simulink library "vmc"  (R2021b)
settings: Solver=VariableStepAuto  StartTime=0.0  StopTime=10.0  RelTol=1e-3
undefined symbols (not defined in the file or in its folder): AVMC_ACCDeltaTqIGain_X_kph, AVMC_ACCDeltaTqIGain_Y_mps2, AVMC_ACCDeltaTqPGain_X_kph, AVMC_ACCDeltaTqPGain_Y_kph, AVMC_ACCLongSteadyCtrl_X_kph, AVMC_AggressJerkPCT4AT_X_kph, AVMC_AggressJerkPCT_X_kph, AVMC_AggressLimitPCT4AT_X_kph, AVMC_AggressLimitPCT_X_kph, AVMC_CCLongSteadyCtrl_X_kph, AVMC_DISCDeltaTqIGain_X_kph, AVMC_DISCDeltaTqIGain_Y_mps2, AVMC_DISCDeltaTqPGain_X_kph, AVMC_DISCDeltaTqPGain_Y_kph, AVMC_DISCTrunAccJerk_X_s, AVMC_DISCTrunAccLimit_X_s, AVMC_ESCRegenOut_X_kph, AVMC_ESCRegenOut_Y_Deg, AVMC_ESCRegenOutEnSpd_X_Deg, AVMC_ISOAccLimit_X_mps, AVMC_ISODecLimit_X_mps, AVMC_ISOJerk_X_mps, AVMC_LatESCRegenOut_X_kph, AVMC_LatESCRegenOut_Y_Deg, AVMC_LongAccDeadZone_X_kph, AVMC_LongAccFiltTsforP2_X_Gps, AVMC_MCPresBaseTq_X_bar, AVMC_MSALongSteadyCtrl_X_kph, AVMC_MSAPedalOvrd2_X_kph, AVMC_MSAPedalOvrd_X_kph, AVMC_MSASpdBand_X_kph, AVMC_MSATqDownEndTq_X_kph, AVMC_MSATqDownTime_X_kph, AVMC_RDCDetectTime_X_kph, AVMC_RDCDetectTime_Y_pct, AVMC_RDCEnSlideRate_X_Deg, AVMC_RearWhlTqRatio_X_Nm, AVMC_RearWhlTqRatio_Y_gps, AVMC_RearWhlTqSlipGain_X_rat, AVMC_RearWhlTqSlipGain_Y_kph, AVMC_SoftJerkPCT_X_kph, AVMC_SoftLimitPCT_X_kph, AVMC_StESCYaw_X_kph, AVMC_StESCYaw_Y_Deg, AVMC_StESCYawCom_X_kph, AVMC_StESCYawCom_Y_Gps, AVMC_TMSpdBaseTq_X_rpm, AVMC_VehHoldBDecMap_X_kph, AVMC_VehHoldDecCtrlTime_X_kph, AVMC_VehHoldMCPPass_X_deg, C_TASK_10MS_S, C_TASK_5MS_S, DEG2RAD, Discrete, ENUM_ACCAVAIL_AVAILABLE, ENUM_ACCCTRLALLOW_ALLOW, ENUM_ADASACCSTA_ACTIVE, ENUM_ADASACCSTA_OVERRIDE, ENUM_ADASACCSTA_SHUTOFF, ENUM_ADASAEBREQ_NOREQUEST ... (+361)
libraries: hcu_lib x63, simulink x60, simulink_extras x3, ctrlSharedLib x3, $bdroot x2
(part 4 of 15)

== system vmc/VMC/VMC/PreConditionCheck ==
  VINP_DriverSeatBeltCmd_flg : Inport
  VBCM_DrDoorSW_flg : Inport  Port=2
  VTQD_GearActualPosn_enum : Inport  Port=3
  VINP_BrkSwSta_flg : Inport  Port=4
  VINP_EPBSta_enum : Inport  Port=5
  VINP_ACCAvail_flg : Inport  Port=6
  VINP_AEBAvail_flg : Inport  Port=7
  VINP_ESCOFFStatus_enum : Inport  Port=8
  VAPS_APSStaSystem_enum : Inport  Port=9
  VTQD_ExternalTqAllow_flg : Inport  Port=10
  VVMC_ACCCtrlAvail_flg : Inport  Port=11
  task_time_s : Inport  Port=12
  VINP_BrkPedalPos_pct : Inport  Port=13
  Cast To Single : DataTypeConversion  OutDataTypeStr=boolean
  Constant : Constant  Value=ENUM_DRDOORSW_CLOSE
  Constant1 : Constant  Value=ENUM_GEARACTUALPOSN_D
  Constant10 : Constant  Value=ENUM_APSSTASYSTEM_ACTIVE
  Constant11 : Constant  Value=ENUM_APSSTASYSTEM_REMOTEACTIVE
  Constant12 : Constant  Value=ENUM_EXTERNALTQALLOW_ALLOW
  Constant13 : Constant  Value=ENUM_ACCCTRLALLOW_ALLOW
  Constant14 : Constant  Value=ENUM_DRDOORSW_CLOSE
  Constant15 : Constant  Value=ENUM_GEARACTUALPOSN_D
  Constant16 : Constant  Value=KVMC_APSSWC_flg
  Constant17 : Constant  Value=ENUM_EPBSTA_RELEASED
  Constant18 : Constant  Value=ENUM_EXTERNALTQALLOW_ALLOW
  Constant{19,21,24,27,30} (5 alike) : Constant  Value=TRUE
  Constant2 : Constant  Value=ENUM_BRKSWSTA_INACTIVE
  Constant{20,23,26,29} (4 alike) : Constant  Value=KVMC_PreCheckAllowTime_s
  Constant{22,25,28,31} (4 alike) : Constant  Value=FALSE
  Constant3 : Constant  Value=ENUM_EPBSTA_RELEASED
  Constant32 : Constant  Value=KVMC_BrkEnBand_pct
  Constant33 : Constant  Value=KVMC_BrkPreCheckSW_flg
  Constant4 : Constant  Value=ENUM_ACCAVAIL_AVAILABLE
  Constant5 : Constant  Value=ENUM_AEBAVAIL_AVAILABLE
  Constant6 : Constant  Value=ENUM_ESCOFFSTATUS_NORMAL
  Constant7 : Constant  Value=ENUM_DRIVERSEATBELTCMD_LAMPOFF
  Constant8 : Constant  Value=ENUM_GEARACTUALPOSN_D
  Constant9 : Constant  Value=ENUM_GEARACTUALPOSN_N
  Logical Operator : Logic  AllPortsSameDT=off  OutDataTypeStr=boolean
  Logical Operator1 : Logic  Inputs=6  AllPortsSameDT=off  OutDataTypeStr=boolean
  Logical Operator2 : Logic  Inputs=3  AllPortsSameDT=off  OutDataTypeStr=boolean
  Logical Operator3 : Logic  Inputs=3  AllPortsSameDT=off  OutDataTypeStr=boolean
  Logical Operator4 : Logic  AllPortsSameDT=off  OutDataTypeStr=boolean
  Logical Operator5 : Logic  Inputs=4  AllPortsSameDT=off  OutDataTypeStr=boolean
  Logical Operator6 : Logic  Operator=OR  AllPortsSameDT=off  OutDataTypeStr=boolean
  NOT{,1..3} (4 alike) : Logic  Operator=NOT  AllPortsSameDT=off  OutDataTypeStr=boolean
  Relational Operator{,1..9,12..15,17..18} (16 alike) : RelationalOperator  Operator===  OutDataTypeStr=boolean  RndMeth=Simplest
  Relational Operator10 : RelationalOperator  Operator=~=  OutDataTypeStr=boolean  RndMeth=Simplest
  Relational Operator11 : RelationalOperator  Operator=~=  OutDataTypeStr=boolean  RndMeth=Simplest
  Relational Operator{16,19..21} (4 alike) : RelationalOperator  OutDataTypeStr=boolean  RndMeth=Simplest
  Relational Operator22 : RelationalOperator  Operator=<=  OutDataTypeStr=boolean  RndMeth=Simplest
  Switch : Switch  Criteria=u2 > Threshold
  Timer{,1..3} (4 alike) : hcu_lib/Basic_Blocks/Timer
  u2 > 0 : Switch  Criteria=u2 > Threshold
  u2 > 0 (1){,1..3} (4 alike) : Switch  Criteria=u2 > Threshold
  VVMC_VMCACCCtrlAvail_flg : Outport
  VVMC_VMCAEBCtrlAvail_flg : Outport  Port=2
  VVMC_VMCCCCtrlAvail_flg : Outport  Port=3
  VVMC_VMCMSACtrlAvail_flg : Outport  Port=4
  wires:
  [task_time_s] -> Timer3/3
  Constant31/1 -> u2 > 0 (1)3/3
  Relational Operator21/1 -> u2 > 0 (1)3/2
  Timer3/1 -> Relational Operator21/1
  Constant29/1 -> Relational Operator21/2, Timer3/4
  Constant30/1 -> u2 > 0 (1)3/1
  Logical Operator5/1 -> NOT3/1, Timer3/1
  NOT3/1 -> Timer3/2
  u2 > 0 (1)3/1 -> [VVMC_VMCMSACtrlAvail_flg]  "VVMC_VMCMSACtrlAvail_flg"
  u2 > 0 (1)2/1 -> [VVMC_VMCCCCtrlAvail_flg]  "VVMC_VMCCCCtrlAvail_flg"
  NOT2/1 -> Timer2/2
  Logical Operator4/1 -> Timer2/1, NOT2/1
  Constant27/1 -> u2 > 0 (1)2/1
  Constant26/1 -> Timer2/4, Relational Operator20/2
  Timer2/1 -> Relational Operator20/1
  Relational Operator20/1 -> u2 > 0 (1)2/2
  Constant28/1 -> u2 > 0 (1)2/3
  [task_time_s] -> Timer2/3
  u2 > 0 (1)1/1 -> [VVMC_VMCACCCtrlAvail_flg]  "VVMC_VMCACCCtrlAvail_flg"
  [task_time_s] -> Timer1/3
  Constant25/1 -> u2 > 0 (1)1/3
  Relational Operator19/1 -> u2 > 0 (1)1/2
  Timer1/1 -> Relational Operator19/1
  Constant23/1 -> Relational Operator19/2, Timer1/4
  Constant24/1 -> u2 > 0 (1)1/1
  Logical Operator2/1 -> NOT1/1, Timer1/1
  NOT1/1 -> Timer1/2
  task_time_s/1 -> [task_time_s]
  u2 > 0 (1)/1 -> [VVMC_VMCAEBCtrlAvail_flg]  "VVMC_VMCAEBCtrlAvail_flg"
  Logical Operator3/1 -> NOT/1, Timer/1
  NOT/1 -> Timer/2
  Constant21/1 -> u2 > 0 (1)/1
  Constant20/1 -> Relational Operator16/2, Timer/4
  Relational Operator16/1 -> u2 > 0 (1)/2
  Timer/1 -> Relational Operator16/1
  [task_time_s] -> Timer/3
  Constant22/1 -> u2 > 0 (1)/3
  Cast To Single/1 -> Logical Operator1/6
  u2 > 0/1 -> Cast To Single/1
  Constant19/1 -> u2 > 0/3
  Constant16/1 -> u2 > 0/2
  Relational Operator5/1 -> Logical Operator3/3
  Relational Operator7/1 -> Logical Operator3/1
  Logical Operator6/1 -> Logical Operator3/2
  Relational Operator8/1 -> Logical Operator6/1
  Relational Operator9/1 -> Logical Operator6/2
  [VTQD_GearActualPosn_enum] -> Relational Operator9/1  "VTQD_GearActualPosn_enum"
  Constant9/1 -> Relational Operator9/2
  Constant8/1 -> Relational Operator8/2
  [VTQD_GearActualPosn_enum] -> Relational Operator8/1  "VTQD_GearActualPosn_enum"
  Constant7/1 -> Relational Operator7/2
  [VINP_DriverSeatBeltCmd_flg] -> Relational Operator7/1
  VINP_DriverSeatBeltCmd_flg/1 -> [VINP_DriverSeatBeltCmd_flg]
  [VVMC_VMCMSACtrlAvail_flg] -> VVMC_VMCMSACtrlAvail_flg/1
  Relational Operator18/1 -> Logical Operator5/4
  Relational Operator17/1 -> Logical Operator5/3
  Relational Operator15/1 -> Logical Operator5/2
  Relational Operator14/1 -> Logical Operator5/1
  Constant18/1 -> Relational Operator18/2
  [VTQD_ExternalTqAllow_flg] -> Relational Operator18/1
  Constant14/1 -> Relational Operator14/2
  [VBCM_DrDoorSW_flg] -> Relational Operator14/1  "VBCM_DrDoorSW_flg"
  Constant15/1 -> Relational Operator15/2
  [VTQD_GearActualPosn_enum] -> Relational Operator15/1  "VTQD_GearActualPosn_enum"
  Constant17/1 -> Relational Operator17/2
  [VINP_EPBSta_enum] -> Relational Operator17/1  "VINP_EPBSta_enum"
  Relational Operator13/1 -> Logical Operator2/2
  [VVMC_ACCCtrlAvail_flg] -> Relational Operator13/1
  Constant13/1 -> Relational Operator13/2
  VVMC_ACCCtrlAvail_flg/1 -> [VVMC_ACCCtrlAvail_flg]
  [VVMC_VMCCCCtrlAvail_flg] -> VVMC_VMCCCCtrlAvail_flg/1
  Relational Operator12/1 -> Logical Operator4/2
  [VTQD_ExternalTqAllow_flg] -> Relational Operator12/1
  Constant12/1 -> Relational Operator12/2
  VTQD_ExternalTqAllow_flg/1 -> [VTQD_ExternalTqAllow_flg]
  [VVMC_VMCACCCtrlAvail_flg] -> VVMC_VMCACCCtrlAvail_flg/1
  [VVMC_VMCAEBCtrlAvail_flg] -> VVMC_VMCAEBCtrlAvail_flg/1
  Logical Operator1/1 -> Logical Operator4/1, Logical Operator2/3
  Relational Operator4/1 -> Logical Operator2/1
  Logical Operator/1 -> u2 > 0/1
  Relational Operator6/1 -> Logical Operator1/5
  Relational Operator3/1 -> Logical Operator1/4
  Switch/1 -> Logical Operator1/3
  Relational Operator1/1 -> Logical Operator1/2
  Relational Operator/1 -> Logical Operator1/1
  Relational Operator11/1 -> Logical Operator/2
  Relational Operator10/1 -> Logical Operator/1
  Constant11/1 -> Relational Operator11/2
  [VAPS_APSStaSystem_enum] -> Relational Operator11/1  "VAPS_APSStaSystem_enum"
  Constant10/1 -> Relational Operator10/2
  [VAPS_APSStaSystem_enum] -> Relational Operator10/1  "VAPS_APSStaSystem_enum"
  Constant6/1 -> Relational Operator6/2
  [VINP_ESCOFFStatus_enum] -> Relational Operator6/1  "VINP_ESCOFFStatus_enum"
  Constant5/1 -> Relational Operator5/2
  [VINP_AEBAvail_flg] -> Relational Operator5/1  "VINP_AEBAvail_flg"
  Constant4/1 -> Relational Operator4/2
  [VINP_ACCAvail_flg] -> Relational Operator4/1  "VINP_ACCAvail_flg"
  [VINP_EPBSta_enum] -> Relational Operator3/1  "VINP_EPBSta_enum"
  Constant3/1 -> Relational Operator3/2
  Constant2/1 -> Relational Operator2/2
  [VINP_BrkSwSta_flg] -> Relational Operator2/1  "VINP_BrkSwSta_flg"
  [VTQD_GearActualPosn_enum] -> Relational Operator1/1  "VTQD_GearActualPosn_enum"
  Constant1/1 -> Relational Operator1/2
  [VBCM_DrDoorSW_flg] -> Relational Operator/1  "VBCM_DrDoorSW_flg"
  Constant/1 -> Relational Operator/2
  VAPS_APSStaSystem_enum/1 -> [VAPS_APSStaSystem_enum]
  VINP_ESCOFFStatus_enum/1 -> [VINP_ESCOFFStatus_enum]
  VINP_AEBAvail_flg/1 -> [VINP_AEBAvail_flg]
  VINP_ACCAvail_flg/1 -> [VINP_ACCAvail_flg]
  VINP_EPBSta_enum/1 -> [VINP_EPBSta_enum]
  VINP_BrkSwSta_flg/1 -> [VINP_BrkSwSta_flg]
  VTQD_GearActualPosn_enum/1 -> [VTQD_GearActualPosn_enum]
  VBCM_DrDoorSW_flg/1 -> [VBCM_DrDoorSW_flg]
  VINP_BrkPedalPos_pct/1 -> [VINP_BrkPedalPos_pct]
  Constant32/1 -> Relational Operator22/2
  Constant33/1 -> Switch/2
  Relational Operator22/1 -> Switch/1
  [VINP_BrkPedalPos_pct] -> Relational Operator22/1
  Relational Operator2/1 -> Switch/3

== system vmc/VMC/VMC/RDC Determination ==
  task_time_s : Inport
  VVMC_ActMaxSlideRate_pct : Inport  Port=2
  VTQD_AfterAvailableTqDemFr_Nm : Inport  Port=3
  VTQD_AfterAvailableTqDemRr_Nm : Inport  Port=4
  VINP_ESCActive_flg : Inport  Port=5
  VINP_SASAngle_Deg : Inport  Port=6
  VINP_LatAccel_Gps : Inport  Port=7
  VINP_VehSpeed_kph : Inport  Port=8
  VINP_YawRate_degps : Inport  Port=9
  VINP_RDCActive_enum : Inport  Port=10
  VINP_DIDGetDynoMode_flg : Inport  Port=11
  RWD : Subsystem
  VVMC_RWDRDCActive_enum : Outport
  VVMC_RDCEnSlideRate_pct : Outport  Port=2
  VVMC_ActStESCYaw_degps : Outport  Port=3
  wires:
  [VINP_YawRate_degps] -> RWD/9(VINP_YawRate_degps)
  VTQD_AfterAvailableTqDemFr_Nm/1 -> [VTQD_AfterAvailableTqDemFr_Nm]
  [VTQD_AfterAvailableTqDemRr_Nm] -> RWD/4(VTQD_AfterAvailableTqDemRr_Nm)
  [VINP_RDCActive_enum] -> RWD/10(VINP_RDCActive_enum)
  [VINP_VehSpeed_kph] -> RWD/8(VINP_VehSpeed_kph)
  [VVMC_RWDRDCActive_enum] -> VVMC_RWDRDCActive_enum/1
  [VINP_LatAccel_Gps] -> RWD/7(VINP_LatAccel_Gps)
  [VVMC_ActMaxSlideRate_pct] -> RWD/2(VVMC_ActMaxSlideRate_pct)
  [VINP_SASAngle_Deg] -> RWD/6(VINP_SASAngle_Deg)
  [task_time_s] -> RWD/1(task_time_s)
  [VTQD_AfterAvailableTqDemFr_Nm] -> RWD/3(VTQD_AfterAvailableTqDemFr_Nm)
  [VINP_ESCActive_flg] -> RWD/5(VINP_ESCActive_flg)
  VINP_RDCActive_enum/1 -> [VINP_RDCActive_enum]
  VINP_SASAngle_Deg/1 -> [VINP_SASAngle_Deg]
  VTQD_AfterAvailableTqDemRr_Nm/1 -> [VTQD_AfterAvailableTqDemRr_Nm]
  task_time_s/1 -> [task_time_s]
  VVMC_ActMaxSlideRate_pct/1 -> [VVMC_ActMaxSlideRate_pct]
  VINP_LatAccel_Gps/1 -> [VINP_LatAccel_Gps]
  VINP_ESCActive_flg/1 -> [VINP_ESCActive_flg]
  VINP_VehSpeed_kph/1 -> [VINP_VehSpeed_kph]
  VINP_YawRate_degps/1 -> [VINP_YawRate_degps]
  RWD/1(VVMC_RWDRDCActive_enum) -> [VVMC_RWDRDCActive_enum]
  RWD/2(VVMC_RDCEnSlideRate_pct) -> [VVMC_RDCEnSlideRate_pct]
  RWD/3(VVMC_ActStESCYaw_Dps) -> [VVMC_ActStESCYaw_degps]
  [VVMC_RDCEnSlideRate_pct] -> VVMC_RDCEnSlideRate_pct/1
  [VVMC_ActStESCYaw_degps] -> VVMC_ActStESCYaw_degps/1
  VINP_DIDGetDynoMode_flg/1 -> [VINP_DIDGetDynoMode_flg]
  [VINP_DIDGetDynoMode_flg] -> RWD/11(VINP_DIDGetDynoMode_flg)

== system vmc/VMC/VMC/SPD2ACC ==
  VVMC_FeatArbitrSta_enum : Inport
  VINP_ADASACCSta_enum : Inport  Port=2
  VVMC_FeatReqSpd_kph : Inport  Port=3
  VVMC_LimitPCT_pct : Inport  Port=4
  VVMC_JerkPCT_pct : Inport  Port=5
  VINP_VehSpeed_kph : Inport  Port=6
  VVMC_MeterIndSpeedForCalcu_kph : Inport  Port=7
  VVMC_SafetyCtrl_flg : Inport  Port=8
  VINP_ACCRequiredAccel_mps2 : Inport  Port=9
  task_time_s : Inport  Port=10
  VVMC_LongAcc_Gps : Inport  Port=11
  VINP_ESCADASSta_enum : Inport  Port=12
  VVMC_LastADASWhlTqReq_Nm : Inport  Port=13
  VTQD_RrEDUAvailBrkRgnTq_Nm : Inport  Port=14
  VVMC_ACCVehHoldReq_flg : Inport  Port=15
  VVMC_EstSlope_Deg : Inport  Port=16
  VVMC_LongAccDeadZone_Gps : Inport  Port=17
  VTQD_FrEDUAvailBrkRgnTq_Nm : Inport  Port=18
  VVMC_ACCLowSpdTqCtrl_flg : Inport  Port=19
  VDSC_DISCTurn_flg : Inport  Port=20
  VINP_GRADE_Deg : Inport  Port=21
  VINP_LFWhlRotDir_enum : Inport  Port=22
  VINP_LRWhlRotDir_enum : Inport  Port=23
  VINP_RFWhlRotDir_enum : Inport  Port=24
  VINP_RRWhlRotDir_enum : Inport  Port=25
  VVMC_ACCObjDist_m : Inport  Port=26
  VINP_MCPressure_bar : Inport  Port=27
  VVMC_AccelTurnHold_flg : Inport  Port=28
  Cast To Boolean : DataTypeConversion  OutDataTypeStr=boolean
  Cast To Boolean1 : DataTypeConversion  OutDataTypeStr=boolean
  Cast To Single : DataTypeConversion  OutDataTypeStr=boolean
  Cast To Single{1..2,4..7,9} (7 alike) : DataTypeConversion  OutDataTypeStr=single
  Cast To Single8 : DataTypeConversion  OutDataTypeStr=uint8
  ISO22179 : Subsystem
  PID : Subsystem
  ReqACCCalcu : Subsystem
  SPD2ACC Active Determination : Subsystem
  VVMC_ACCRequiredAccel_mps2 : Outport
  VVMC_DISCReqAcc_mps2 : Outport  Port=2
  VVMC_FeatArbitrFinal_enum : Outport  Port=3
  VVMC_SPD2ACCAct_flg : Outport  Port=4
  VVMC_AccCalcuPID_mps2 : Outport  Port=5
  VVMC_ISOAccLimit_mps2 : Outport  Port=6
  VVMC_ISODecLimit_mps2 : Outport  Port=7
  VVMC_ISOJerkLimit_mps3 : Outport  Port=8
  VVMC_VehHoldReq_flg : Outport  Port=9
  VVMC_ActACCRequiredAccel_mps2 : Outport  Port=10
  VVMC_VehHoldDecCtrlHEnd_flg : Outport  Port=11
  wires:
  [task_time_s] -> ReqACCCalcu/13(task_time_s)
  task_time_s/1 -> [task_time_s]
  [VINP_VehSpeed_kph] -> PID/3(VINP_VehSpeed_kph)
  VINP_VehSpeed_kph/1 -> [VINP_VehSpeed_kph]
  [VVMC_ISOJerkLimit_mps3] -> VVMC_ISOJerkLimit_mps3/1
  [VVMC_ISODecLimit_mps2] -> VVMC_ISODecLimit_mps2/1
  [VVMC_ISOAccLimit_mps2] -> VVMC_ISOAccLimit_mps2/1
  [VVMC_AccCalcuPID_mps2] -> VVMC_AccCalcuPID_mps2/1
  [VVMC_SPD2ACCAct_flg] -> VVMC_SPD2ACCAct_flg/1
  [VVMC_FeatReqSpd_kph] -> ReqACCCalcu/12(VVMC_FeatReqSpd_kph)
  [VVMC_MeterIndSpeedForCalcu_kph] -> ReqACCCalcu/11(VVMC_MeterIndSpeedForCalcu_kph)
  [VINP_ADASACCSta_enum] -> ReqACCCalcu/10(VINP_ADASACCSta_enum)
  VINP_ADASACCSta_enum/1 -> [VINP_ADASACCSta_enum]
  [VVMC_ActACCRequiredAccel_mps2] -> VVMC_DISCReqAcc_mps2/1  "VVMC_DISCReqAcc_mps2"
  [VVMC_FeatArbitrFinal_enum] -> VVMC_FeatArbitrFinal_enum/1
  Cast To Single8/1 -> [VVMC_FeatArbitrFinal_enum]  "VVMC_FeatArbitrFinal_enum"
  ReqACCCalcu/2(VVMC_FeatArbitrFinal_enum) -> Cast To Single8/1
  [VVMC_FeatArbitrSta_enum] -> ReqACCCalcu/9(VVMC_FeatArbitrSta_enum)
  [VINP_ACCRequiredAccel_mps2] -> ReqACCCalcu/8(VINP_ACCRequiredAccel_mps2)
  VINP_ACCRequiredAccel_mps2/1 -> [VINP_ACCRequiredAccel_mps2]
  VVMC_SafetyCtrl_flg/1 -> [VVMC_SafetyCtrl_flg]
  [VVMC_SafetyCtrl_flg] -> ReqACCCalcu/7(VVMC_SafetyCtrl_flg)
  Cast To Single7/1 -> [VVMC_ACCRequiredAccel_mps2]  "VVMC_ACCRequiredAccel_mps2"
  Cast To Single6/1 -> [VVMC_ISOJerkLimit_mps3]  "VVMC_ISOJerkLimit_mps3"
  Cast To Single5/1 -> [VVMC_ISODecLimit_mps2]  "VVMC_ISODecLimit_mps2"
  Cast To Single4/1 -> [VVMC_ISOAccLimit_mps2]  "VVMC_ISOAccLimit_mps2"
  Cast To Single2/1 -> [VVMC_MeterSpdCalcu_mps]  "VVMC_MeterSpdCalcu_mps"
  Cast To Single1/1 -> [VVMC_AccCalcuPID_mps2]  "VVMC_AccCalcuPID_mps2"
  Cast To Single/1 -> [VVMC_SPD2ACCAct_flg]  "VVMC_SPD2ACCAct_flg"
  [VVMC_ACCRequiredAccel_mps2] -> VVMC_ACCRequiredAccel_mps2/1
  ReqACCCalcu/1("VVMC_ACCRequiredAccel_mps2 ") -> Cast To Single7/1
  [VVMC_SPD2ACCAct_flg] -> ReqACCCalcu/6(VVMC_SPD2ACCAct_flg)
  PID/2(VVMC_MeterSpdCalcu_mps) -> Cast To Single2/1
  PID/1(VVMC_AccCalcuPID_mps2) -> Cast To Single1/1
  [VVMC_FeatReqSpd_kph] -> PID/2(VVMC_FeatReqSpd_kph)
  [VVMC_MeterIndSpeedForCalcu_kph] -> PID/4(VVMC_MeterIndSpeedForCalcu_kph)
  [VVMC_SPD2ACCAct_flg] -> PID/1(VVMC_SPD2ACCAct_flg)
  ISO22179/3(VVMC_ISOJerkLimit_mps3) -> Cast To Single6/1
  [VVMC_MeterSpdCalcu_mps] -> ISO22179/1(VVMC_MeterSpdCalcu_mps)
  ISO22179/2(VVMC_ISODecLimit_mps2) -> Cast To Single5/1
  ISO22179/1(VVMC_ISOAccLimit_mps2) -> Cast To Single4/1
  [VVMC_LimitPCT_pct] -> ISO22179/2(VVMC_LimitPCT_pct)
  SPD2ACC Active Determination/1(VVMC_SPD2ACCAct_flg) -> Cast To Single/1
  [VVMC_FeatArbitrSta_enum] -> SPD2ACC Active Determination/1(VVMC_FeatArbitrSta_enum)
  VVMC_FeatArbitrSta_enum/1 -> [VVMC_FeatArbitrSta_enum]
  VVMC_MeterIndSpeedForCalcu_kph/1 -> [VVMC_MeterIndSpeedForCalcu_kph]
  VVMC_LimitPCT_pct/1 -> [VVMC_LimitPCT_pct]
  VVMC_JerkPCT_pct/1 -> [VVMC_JerkPCT_pct]
  VVMC_FeatReqSpd_kph/1 -> [VVMC_FeatReqSpd_kph]
  [VVMC_JerkPCT_pct] -> ReqACCCalcu/3(VVMC_JerkPCT_pct)
  [VVMC_ISOJerkLimit_mps3] -> ReqACCCalcu/2(VVMC_ISOJerkLimit_mps3)
  [VVMC_AccCalcuPID_mps2] -> ReqACCCalcu/1(VVMC_AccCalcuPID_mps2)
  [VVMC_ISOAccLimit_mps2] -> ReqACCCalcu/4(VVMC_ISOAccLimit_mps2)
  [VVMC_ISODecLimit_mps2] -> ReqACCCalcu/5(VVMC_ISODecLimit_mps2)
  [VINP_VehSpeed_kph] -> ReqACCCalcu/14(VINP_VehSpeed_kph)
  [VVMC_LongAcc_Gps] -> ReqACCCalcu/15(VVMC_LongAcc_Gps)
  VVMC_LongAcc_Gps/1 -> [VVMC_LongAcc_Gps]
  [VTQD_RrEDUAvailBrkRgnTq_Nm] -> ReqACCCalcu/18(VTQD_RrEDUAvailBrkRgnTq_Nm)
  [VVMC_LastADASWhlTqReq_Nm] -> ReqACCCalcu/17(VVMC_LastADASWhlTqReq_Nm)
  [VINP_ESCADASSta_enum] -> ReqACCCalcu/16(VINP_ESCADASSta_enum)
  Cast To Boolean/1 -> [VVMC_VehHoldReq_flg]  "VVMC_VehHoldReq_flg"
  Cast To Single9/1 -> [VVMC_ActACCRequiredAccel_mps2]  "VVMC_ActACCRequiredAccel_mps2"
  ReqACCCalcu/4(VVMC_ActACCRequiredAccel_mps2) -> Cast To Single9/1
  ReqACCCalcu/3(VVMC_VehHoldReq_flg) -> Cast To Boolean/1
  VTQD_RrEDUAvailBrkRgnTq_Nm/1 -> [VTQD_RrEDUAvailBrkRgnTq_Nm]
  VINP_ESCADASSta_enum/1 -> [VINP_ESCADASSta_enum]
  VVMC_LastADASWhlTqReq_Nm/1 -> [VVMC_LastADASWhlTqReq_Nm]
  [VVMC_ActACCRequiredAccel_mps2] -> VVMC_ActACCRequiredAccel_mps2/1
  [VVMC_VehHoldReq_flg] -> VVMC_VehHoldReq_flg/1  "VVMC_VehHoldReq_flg"
  VVMC_ACCVehHoldReq_flg/1 -> [VVMC_ACCVehHoldReq_flg]
  [VVMC_ACCVehHoldReq_flg] -> ReqACCCalcu/19(VVMC_ACCVehHoldReq_flg)
  VVMC_EstSlope_Deg/1 -> [VVMC_EstSlope_Deg]
  [VVMC_EstSlope_Deg] -> ReqACCCalcu/20(VVMC_EstSlope_Deg)
  VVMC_LongAccDeadZone_Gps/1 -> [VVMC_LongAccDeadZone_Gps]
  [VVMC_LongAccDeadZone_Gps] -> ReqACCCalcu/21(VVMC_LongAccDeadZone_Gps)
  ReqACCCalcu/5(VVMC_VehHoldDecCtrlHEnd_flg) -> Cast To Boolean1/1
  Cast To Boolean1/1 -> [VVMC_VehHoldDecCtrlHEnd_flg]
  [VVMC_VehHoldDecCtrlHEnd_flg] -> VVMC_VehHoldDecCtrlHEnd_flg/1
  VTQD_FrEDUAvailBrkRgnTq_Nm/1 -> [VTQD_FrEDUAvailBrkRgnTq_Nm]
  [VTQD_FrEDUAvailBrkRgnTq_Nm] -> ReqACCCalcu/22(VTQD_FrEDUAvailBrkRgnTq_Nm)
  VVMC_ACCLowSpdTqCtrl_flg/1 -> [VVMC_ACCLowSpdTqCtrl_flg]
  [VVMC_ACCLowSpdTqCtrl_flg] -> ReqACCCalcu/23(VVMC_ACCLowSpdTqCtrl_flg)
  VDSC_DISCTurn_flg/1 -> [VDSC_DISCTurn_flg]
  [VDSC_DISCTurn_flg] -> ReqACCCalcu/24(VDSC_DISCTurn_flg)
  VINP_GRADE_Deg/1 -> [VINP_GRADE_Deg]
  [VINP_GRADE_Deg] -> ReqACCCalcu/25(VINP_GRADE_Deg)
  VINP_LRWhlRotDir_enum/1 -> [VINP_LRWhlRotDir_enum]
  VINP_RFWhlRotDir_enum/1 -> [VINP_RFWhlRotDir_enum]
  VINP_LFWhlRotDir_enum/1 -> [VINP_LFWhlRotDir_enum]
  VINP_RRWhlRotDir_enum/1 -> [VINP_RRWhlRotDir_enum]
  [VINP_RRWhlRotDir_enum] -> ReqACCCalcu/29(VINP_RRWhlRotDir_enum)
  [VINP_RFWhlRotDir_enum] -> ReqACCCalcu/28(VINP_RFWhlRotDir_enum)
  [VINP_LRWhlRotDir_enum] -> ReqACCCalcu/27(VINP_LRWhlRotDir_enum)
  [VINP_LFWhlRotDir_enum] -> ReqACCCalcu/26(VINP_LFWhlRotDir_enum)
  VVMC_ACCObjDist_m/1 -> [VVMC_ACCObjDist_m]
  [VVMC_ACCObjDist_m] -> ReqACCCalcu/30(VVMC_ACCObjDist_m)
  VINP_MCPressure_bar/1 -> [VINP_MCPressure_bar]
  [VINP_MCPressure_bar] -> ReqACCCalcu/31(VINP_MCPressure_bar)
  VVMC_AccelTurnHold_flg/1 -> [VVMC_AccelTurnHold_flg]
  [VVMC_AccelTurnHold_flg] -> ReqACCCalcu/32(VVMC_AccelTurnHold_flg)

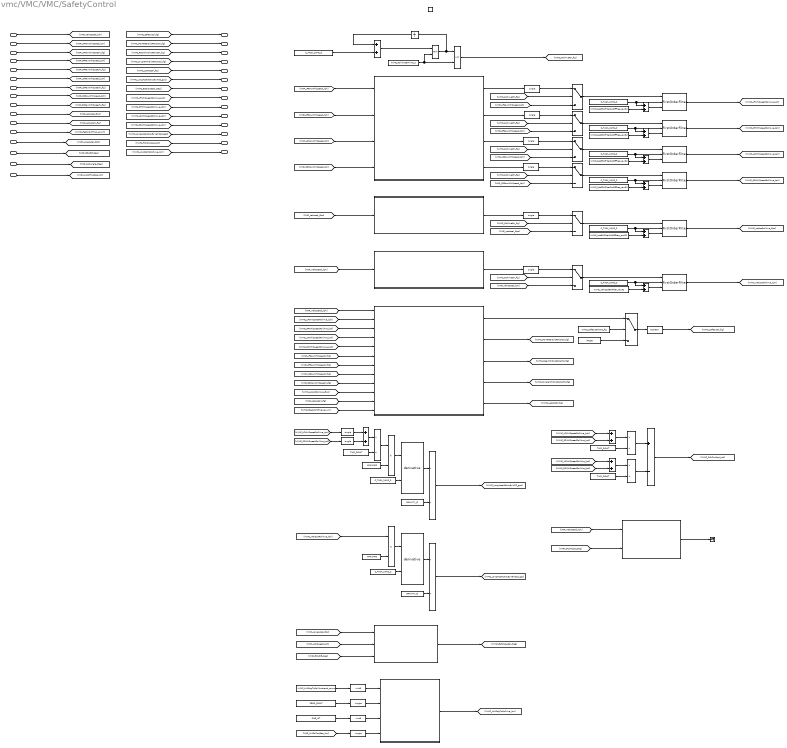
== system vmc/VMC/VMC/SafetyControl ==
  VINP_VehSpeed_kph : Inport
  VINP_LFRawWhlSpeed_kph : Inport  Port=2
  VINP_LFRawWhlSpeedV_flg : Inport  Port=3
  VINP_RFRawWhlSpeed_kph : Inport  Port=4
  VINP_RFRawWhlSpeedV_flg : Inport  Port=5
  VINP_LRRawWhlSpeed_kph : Inport  Port=6
  VINP_LRRawWhlSpeedV_flg : Inport  Port=7
  VINP_RRRawWhlSpeed_kph : Inport  Port=8
  VINP_RRRawWhlSpeedV_flg : Inport  Port=9
  VINP_LatAccel_Gps : Inport  Port=10
  VINP_LatAccelV_flg : Inport  Port=11
  VVMC_FeatArbitrFinal_enum : Inport  Port=12
  VINP_LongAccel_Gps : Inport  Port=13
  VINP_GRADE_deg : Inport  Port=14
  VINP_SASAngle_Deg : Inport  Port=15
  VINP_LKAStrToqReq_Nm : Inport  Port=16
  function : TriggerPort  TriggerType=function-call  VariantControl=(inherit)
  Add{,1..9} (10 alike) : Sum
  Add10 : Sum  Inputs=+-
  Cast To Single{,1..4,6..8,10..11} (10 alike) : DataTypeConversion  OutDataTypeStr=single
  Cast To Single12 : DataTypeConversion  OutDataTypeStr=uint8
  Cast To Single5 : DataTypeConversion  OutDataTypeStr=boolean
  Cast To Single9 : DataTypeConversion  OutDataTypeStr=uint8
  Constant : Constant  Value=FALSE
  Constant1 : Constant  Value=KVMC_SafetyCtrlSWC_flg
  Constant{4,6..10,16,22,26} (9 alike) : Constant  Value=C_TASK_10MS_S
  Constant{11..13,15} (4 alike) : Constant  Value=KVMC_SpdBWFilterCutOffFreq_raw32
  Constant14 : Constant  Value=GRAVITY_G
  Constant17 : Constant  Value=KVMC_AccBWFilterCutOffFreq_raw32
  Constant18 : Constant  Value=TWO_FLOAT
  Constant19 : Constant  Value=TWO_FLOAT
  Constant2 : Constant  Value=TWO_FLOAT
  Constant20 : Constant  Value=ZERO_FLOAT
  Constant21 : Constant  Value=ONE_INT
  Constant23 : Constant  Value=KVMC_VehSpdBWFilter_raw32
  Constant24 : Constant  Value=GRAVITY_G
  Constant25 : Constant  Value=KPH2MPS
  Constant27 : Constant  Value=KVMC_LKAStrgTqRollAveLevel_enum
  Constant3 : Constant  Value=KPH2MPS
  Constant5 : Constant  Value=KVMC_RollAveEnTime_s
  Divide{,3..6} (5 alike) : Product  Inputs=*/
  Divide1 : Product  Inputs=**
  Divide2 : Product  Inputs=**
  Estimate Slope : Subsystem
  FirstOrderFilter{,1..4,6} (6 alike) : hcu_lib/Basic_Blocks/FirstOrderFilter
  LKAStrgTqRollingAverage : Stateflow chart  TreatAsAtomicUnit=on
  LatAccRollingAverage : Subsystem
  Lateral_Module : Subsystem
  Min1 : MinMax  Inputs=2
  Relational Operator : RelationalOperator  OutDataTypeStr=boolean  RndMeth=Simplest
  SafetyControlJudgement : Subsystem
  Terminator : Terminator
  VehSpdRollingAverage : Subsystem
  WheelSpeedRollingAverage : Subsystem
  derivative : hcu_lib/Basic_Blocks/derivative
  derivative1 : hcu_lib/Basic_Blocks/derivative
  initial: 0 : UnitDelay  SampleTime=-1  HasFrameUpgradeWarning=on
  u2 > 0 : Switch  Criteria=u2 > Threshold
  u2 > 0 (1){,1..4,6} (6 alike) : Switch  Criteria=u2 > Threshold
  VVMC_SafetyCtrl_flg : Outport
  VVMC_FrontRearSlipRatioCtrl_flg : Outport  Port=2
  VVMC_RearWhlSlipRatioCtrl_flg : Outport  Port=3
  VVMC_SingleWhlSlipRatioCtrl_flg : Outport  Port=4
  VVMC_LatAccCtrl_flg : Outport  Port=5
  VVMC_LongAccelCalcuByWSS_gps : Outport  Port=6
  VVMC_EstSlope_Deg : Outport  Port=7
  VVMC_LFWhlSpeedRollAve_kph : Outport  Port=8
  VVMC_RFWhlSpeedRollAve_kph : Outport  Port=9
  VVMC_LRWhlSpeedRollAve_kph : Outport  Port=10
  VVMC_RRWhlSpeedRollAve_kph : Outport  Port=11
  VVMC_LongAccelCalcuByVehSpd_gps : Outport  Port=12
  VVMC_FrRrSlipSpd_kph : Outport  Port=13
  VVMC_LKAStrgTqRollAve_Nm : Outport  Port=14
  wires:
  WheelSpeedRollingAverage/4(VVMC_RRWhlSpeedRollAve_kph) -> Cast To Single3/1
  [VINP_LRRawWhlSpeed_kph] -> WheelSpeedRollingAverage/3(VINP_LRRawWhlSpeed_kph)
  FirstOrderFilter/1 -> [VVMC_RRWhlSpeedRollAve_kph]  "VVMC_RRWhlSpeedRollAve_kph"
  [VVMC_LatAccRollAve_Gps] -> SafetyControlJudgement/10(VVMC_LatAccRollAve_Gps)
  [VVMC_SingleWhlSlipRatioCtrl_flg] -> VVMC_SingleWhlSlipRatioCtrl_flg/1
  VINP_LFRawWhlSpeed_kph/1 -> [VINP_LFRawWhlSpeed_kph]
  SafetyControlJudgement/2(VVMC_FrontRearSlipRatioCtrl_flg) -> [VVMC_FrontRearSlipRatioCtrl_flg]
  SafetyControlJudgement/5(VVMC_LatAccCtrl_flg) -> [VVMC_LatAccCtrl_flg]
  [VINP_RFRawWhlSpeed_kph] -> WheelSpeedRollingAverage/2(VINP_RFRawWhlSpeed_kph)
  Constant3/1 -> Divide1/2
  WheelSpeedRollingAverage/2(VVMC_RFWhlSpeedRollAve_kph) -> Cast To Single1/1
  Divide/1 -> Divide1/1
  FirstOrderFilter3/1 -> [VVMC_LFWhlSpeedRollAve_kph]  "VVMC_LFWhlSpeedRollAve_kph"
  [VINP_LatAccelV_flg] -> SafetyControlJudgement/11(VINP_LatAccelV_flg)
  Constant14/1 -> Divide3/2
  [VINP_LFRawWhlSpeedV_flg] -> SafetyControlJudgement/6(VINP_LFRawWhlSpeedV_flg)
  VINP_RRRawWhlSpeed_kph/1 -> [VINP_RRRawWhlSpeed_kph]
  [VINP_LatAccel_Gps] -> LatAccRollingAverage/1(VINP_LatAccel_Gps)
  derivative/1 -> Divide3/1
  LatAccRollingAverage/1(VVMC_LatAccRollAve_Gps) -> Cast To Single4/1
  VINP_LatAccel_Gps/1 -> [VINP_LatAccel_Gps]
  WheelSpeedRollingAverage/1(VVMC_LFWhlSpeedRollAve_kph) -> Cast To Single/1
  SafetyControlJudgement/4(VVMC_SingleWhlSlipRatioCtrl_flg) -> [VVMC_SingleWhlSlipRatioCtrl_flg]
  Divide3/1 -> [VVMC_LongAccelCalcuByWSS_gps]  "VVMC_LongAccelCalcuByWSS_gps"
  [VVMC_LatAccCtrl_flg] -> VVMC_LatAccCtrl_flg/1
  [VINP_RFRawWhlSpeedV_flg] -> SafetyControlJudgement/7(VINP_RFRawWhlSpeedV_flg)
  Constant1/1 -> u2 > 0/2
  VINP_LRRawWhlSpeed_kph/1 -> [VINP_LRRawWhlSpeed_kph]
  [VVMC_LongAccelCalcuByWSS_gps] -> VVMC_LongAccelCalcuByWSS_gps/1  "VVMC_LongAccelCalcuByWSS_gps"
  FirstOrderFilter4/1 -> [VVMC_LatAccRollAve_Gps]  "VVMC_LatAccRollAve_Gps"
  u2 > 0/1 -> Cast To Single5/1
  [VVMC_RearWhlSlipRatioCtrl_flg] -> VVMC_RearWhlSlipRatioCtrl_flg/1
  VINP_RRRawWhlSpeedV_flg/1 -> [VINP_RRRawWhlSpeedV_flg]
  [VVMC_LRWhlSpeedRollAve_kph] -> SafetyControlJudgement/4(VVMC_LRWhlSpeedRollAve_kph)
  [VINP_RRRawWhlSpeed_kph] -> WheelSpeedRollingAverage/4(VINP_RRRawWhlSpeed_kph)
  [VVMC_RFWhlSpeedRollAve_kph] -> Cast To Single7/1
  [VVMC_RRWhlSpeedRollAve_kph] -> SafetyControlJudgement/5(VVMC_RRWhlSpeedRollAve_kph)
  WheelSpeedRollingAverage/3(VVMC_LRWhlSpeedRollAve_kph) -> Cast To Single2/1
  [VVMC_LFWhlSpeedRollAve_kph] -> Cast To Single6/1
  SafetyControlJudgement/3(VVMC_RearWhlSlipRatioCtrl_flg) -> [VVMC_RearWhlSlipRatioCtrl_flg]
  VINP_LatAccelV_flg/1 -> [VINP_LatAccelV_flg]
  [VINP_LFRawWhlSpeed_kph] -> WheelSpeedRollingAverage/1(VINP_LFRawWhlSpeed_kph)
  VINP_LFRawWhlSpeedV_flg/1 -> [VINP_LFRawWhlSpeedV_flg]
  [VVMC_FeatArbitrFinal_enum] -> SafetyControlJudgement/12(VVMC_FeatArbitrFinal_enum)
  SafetyControlJudgement/1(VVMC_SafetyCtrl_flg) -> u2 > 0/1
  [VINP_RRRawWhlSpeedV_flg] -> SafetyControlJudgement/9(VINP_RRRawWhlSpeedV_flg)
  [VINP_LRRawWhlSpeedV_flg] -> SafetyControlJudgement/8(VINP_LRRawWhlSpeedV_flg)
  VVMC_FeatArbitrFinal_enum/1 -> [VVMC_FeatArbitrFinal_enum]
  [VINP_VehSpeed_kph] -> SafetyControlJudgement/1(VINP_VehSpeed_kph)
  VINP_LRRawWhlSpeedV_flg/1 -> [VINP_LRRawWhlSpeedV_flg]
  VINP_VehSpeed_kph/1 -> [VINP_VehSpeed_kph]
  Constant2/1 -> Divide/2
  [VVMC_SafetyCtrl_flg] -> VVMC_SafetyCtrl_flg/1
  FirstOrderFilter2/1 -> [VVMC_RFWhlSpeedRollAve_kph]  "VVMC_RFWhlSpeedRollAve_kph"
  [VVMC_LFWhlSpeedRollAve_kph] -> SafetyControlJudgement/2(VVMC_LFWhlSpeedRollAve_kph)
  [VVMC_FrontRearSlipRatioCtrl_flg] -> VVMC_FrontRearSlipRatioCtrl_flg/1
  Divide1/1 -> derivative/1
  Cast To Single5/1 -> [VVMC_SafetyCtrl_flg]  "VVMC_SafetyCtrl_flg"
  VINP_RFRawWhlSpeed_kph/1 -> [VINP_RFRawWhlSpeed_kph]
  Add/1 -> Divide/1
  [VVMC_RFWhlSpeedRollAve_kph] -> SafetyControlJudgement/3(VVMC_RFWhlSpeedRollAve_kph)
  FirstOrderFilter1/1 -> [VVMC_LRWhlSpeedRollAve_kph]  "VVMC_LRWhlSpeedRollAve_kph"
  Constant/1 -> u2 > 0/3
  VINP_RFRawWhlSpeedV_flg/1 -> [VINP_RFRawWhlSpeedV_flg]
  initial: 0/1 -> Add2/1
  Constant5/1 -> Min1/2, Relational Operator/2
  Constant6/1 -> Add2/2
  Add2/1 -> Min1/1
  Relational Operator/1 -> [VVMC_RollAveEn_flg]  "VVMC_RollAveEn_flg"
  u2 > 0 (1)2/1 -> FirstOrderFilter1/1
  u2 > 0 (1)/1 -> FirstOrderFilter3/1
  [VINP_RFRawWhlSpeed_kph] -> u2 > 0 (1)1/3
  [VINP_LRRawWhlSpeed_kph] -> u2 > 0 (1)2/3
  [VVMC_RollAveEn_flg] -> u2 > 0 (1)3/2
  [VVMC_RollAveEn_flg] -> u2 > 0 (1)/2
  [VINP_LFRawWhlSpeed_kph] -> u2 > 0 (1)/3
  Cast To Single/1 -> u2 > 0 (1)/1
  [VINP_RRRawWhlSpeed_kph] -> u2 > 0 (1)3/3
  u2 > 0 (1)1/1 -> FirstOrderFilter2/1
  [VVMC_RollAveEn_flg] -> u2 > 0 (1)1/2
  Cast To Single2/1 -> u2 > 0 (1)2/1
  Cast To Single1/1 -> u2 > 0 (1)1/1
  u2 > 0 (1)3/1 -> FirstOrderFilter/1
  Cast To Single3/1 -> u2 > 0 (1)3/1
  [VVMC_RollAveEn_flg] -> u2 > 0 (1)2/2
  Constant7/1 -> Add3/1, FirstOrderFilter3/2
  Constant8/1 -> FirstOrderFilter2/2, Add4/1
  Constant9/1 -> Add5/1, FirstOrderFilter1/2
  Constant10/1 -> FirstOrderFilter/2, Add6/1
  Add3/1 -> FirstOrderFilter3/3
  Constant11/1 -> Add3/2
  Constant12/1 -> Add4/2
  Add4/1 -> FirstOrderFilter2/3
  Constant13/1 -> Add5/2
  Add5/1 -> FirstOrderFilter1/3
  Constant15/1 -> Add6/2
  Add6/1 -> FirstOrderFilter/3
  [VVMC_RollAveEn_flg] -> u2 > 0 (1)4/2
  Cast To Single4/1 -> u2 > 0 (1)4/1
  [VINP_LatAccel_Gps] -> u2 > 0 (1)4/3
  Add7/1 -> FirstOrderFilter4/3
  Constant17/1 -> Add7/2
  Constant16/1 -> FirstOrderFilter4/2, Add7/1
  u2 > 0 (1)4/1 -> FirstOrderFilter4/1
  Cast To Single6/1 -> Add/1
  Cast To Single7/1 -> Add/2
  Constant4/1 -> derivative/2
  [VINP_LongAccel_Gps] -> Estimate Slope/1(VINP_LongAccel_Gps)
  [VINP_GRADE_deg] -> Estimate Slope/3(VINP_GRADE_deg)
  [VINP_VehSpeed_kph] -> Estimate Slope/2(VINP_VehSpeed_kph)
  Estimate Slope/1(VVMC_EstSlope_Deg) -> [VVMC_EstSlopeCal_Deg]
  VINP_LongAccel_Gps/1 -> [VINP_LongAccel_Gps]
  VINP_GRADE_deg/1 -> [VINP_GRADE_deg]
  [VVMC_EstSlopeCal_Deg] -> VVMC_EstSlope_Deg/1
  [VVMC_RRWhlSpeedRollAve_kph] -> VVMC_RRWhlSpeedRollAve_kph/1  "VVMC_RRWhlSpeedRollAve_kph"
  [VVMC_LRWhlSpeedRollAve_kph] -> VVMC_LRWhlSpeedRollAve_kph/1  "VVMC_LRWhlSpeedRollAve_kph"
  [VVMC_RFWhlSpeedRollAve_kph] -> VVMC_RFWhlSpeedRollAve_kph/1  "VVMC_RFWhlSpeedRollAve_kph"
  [VVMC_LFWhlSpeedRollAve_kph] -> VVMC_LFWhlSpeedRollAve_kph/1  "VVMC_LFWhlSpeedRollAve_kph"
  [VINP_VehSpeed_kph] -> VehSpdRollingAverage/1(VINP_VehSpeed_kph)
  Add8/1 -> FirstOrderFilter6/3
  Constant23/1 -> Add8/2
  Constant22/1 -> Add8/1, FirstOrderFilter6/2
  Cast To Single8/1 -> u2 > 0 (1)6/1
  u2 > 0 (1)6/1 -> FirstOrderFilter6/1
  [VINP_VehSpeed_kph] -> u2 > 0 (1)6/3
  [VVMC_RollAveEn_flg] -> u2 > 0 (1)6/2
  FirstOrderFilter6/1 -> [VVMC_VehSpdRollAve_kph]  "VVMC_VehSpdRollAve_kph"
  VehSpdRollingAverage/1(VVMC_VehSpdRollAve_kph) -> Cast To Single8/1
  Constant26/1 -> derivative1/2
  derivative1/1 -> Divide4/1
  Constant24/1 -> Divide4/2
  Constant25/1 -> Divide2/2
  [VVMC_VehSpdRollAve_kph] -> Divide2/1
  Divide2/1 -> derivative1/1
  Divide4/1 -> [VVMC_LongAccelCalcuByVehSpd_gps]  "VVMC_LongAccelCalcuByVehSpd_gps"
  [VVMC_LongAccelCalcuByVehSpd_gps] -> VVMC_LongAccelCalcuByVehSpd_gps/1  "VVMC_LongAccelCalcuByVehSpd_gps"
  [VVMC_LFWhlSpeedRollAve_kph] -> Add1/1
  [VVMC_RFWhlSpeedRollAve_kph] -> Add1/2
  Constant18/1 -> Divide5/2
  [VVMC_LRWhlSpeedRollAve_kph] -> Add9/1
  [VVMC_RRWhlSpeedRollAve_kph] -> Add9/2
  Constant19/1 -> Divide6/2
  Add9/1 -> Divide6/1
  Add1/1 -> Divide5/1
  Divide6/1 -> Add10/2
  Divide5/1 -> Add10/1
  Add10/1 -> [VVMC_FrRrSlipSpd_kph]  "VVMC_FrRrSlipSpd_kph"
  [VVMC_FrRrSlipSpd_kph] -> VVMC_FrRrSlipSpd_kph/1
  [VINP_SASAngle_Deg] -> Lateral_Module/2(VINP_SASAngle_deg)
  [VINP_VehSpeed_kph] -> Lateral_Module/1(VINP_VehSpeed_kph)
  VINP_SASAngle_Deg/1 -> [VINP_SASAngle_Deg]
  Lateral_Module/1(VVMC_TheoYawRate_degps) -> Terminator/1
  Min1/1 -> initial: 0/1, Relational Operator/1
  Constant27/1 -> Cast To Single9/1
  Cast To Single10/1 -> LKAStrgTqRollingAverage/2(ZERO_FLOAT)
  Cast To Single12/1 -> LKAStrgTqRollingAverage/3(ONE_INT)
  Cast To Single9/1 -> LKAStrgTqRollingAverage/1(KVMC_LKAStrgTqRollAveLevel_enum)
  [VINP_LKAStrToqReq_Nm] -> Cast To Single11/1
  Constant20/1 -> Cast To Single10/1
  Cast To Single11/1 -> LKAStrgTqRollingAverage/4(VINP_LKAStrToqReq_Nm)
  Constant21/1 -> Cast To Single12/1
  LKAStrgTqRollingAverage/1(VVMC_LKAStrgTqRollAve_Nm) -> [VVMC_LKAStrgTqRollAve_Nm]
  [VVMC_LKAStrgTqRollAve_Nm] -> VVMC_LKAStrgTqRollAve_Nm/1
  VINP_LKAStrToqReq_Nm/1 -> [VINP_LKAStrToqReq_Nm]

== system vmc/VMC/VMC/Slide Rate  Calculation ==
  VINP_LFRawWhlSpeed_kph : Inport
  VINP_RFRawWhlSpeed_kph : Inport  Port=2
  VINP_LRRawWhlSpeed_kph : Inport  Port=3
  VINP_RRRawWhlSpeed_kph : Inport  Port=4
  VINP_VehSpeed_kph : Inport  Port=5
  VINP_BrkPedalPos_pct : Inport  Port=6
  VINP_BrkSwSta_flg : Inport  Port=7
  VINP_LongAccel_Gps : Inport  Port=8
  VVMC_LongAcc_Gps : Inport  Port=9
  task_time_s : Inport  Port=10
  VTQD_AfterAvailableTqDemFr_Nm : Inport  Port=11
  VTQD_AfterAvailableTqDemRr_Nm : Inport  Port=12
  VTQD_EquivAccPedalSWSta_flg : Inport  Port=13
  VTQD_GearActualPosn_enum : Inport  Port=14
  4Wheel Calculation : Subsystem
  Alternative Wheel Slide Calculation : Subsystem
  Coordination : Subsystem
  Partial Wheel Calculation : Subsystem
  VVMC_RawWhlSpdSlideRate_pct : Outport
  VVMC_LFWhlSpdSlideRate_pct : Outport  Port=2
  VVMC_RFWhlSpdSlideRate_pct : Outport  Port=3
  VVMC_LRWhlSpdSlideRate_pct : Outport  Port=4
  VVMC_RRWhlSpdSlideRate_pct : Outport  Port=5
  VVMC_LF4WhlSpdSlideRate_pct : Outport  Port=6
  VVMC_RF4WhlSpdSlideRate_pct : Outport  Port=7
  VVMC_LR4WhlSpdSlideRate_pct : Outport  Port=8
  VVMC_RR4WhlSpdSlideRate_pct : Outport  Port=9
  VVMC_PredictVehSpd_kph : Outport  Port=10
  VVMC_4WhlSpdSlideRate_pct : Outport  Port=11
  VVMC_ActMaxSlideRate_pct : Outport  Port=12
  VVMC_ActLFSlideRate_pct : Outport  Port=13
  VVMC_ActRFSlideRate_pct : Outport  Port=14
  VVMC_ActLRSlideRate_pct : Outport  Port=15
  VVMC_ActRRSlideRate_pct : Outport  Port=16
  VVMC_AltLWhlSlideRate_pct : Outport  Port=17
  VVMC_AltRWhlSlideRate_pct : Outport  Port=18
  VVMC_AltWhlSlideRate_pct : Outport  Port=19
  wires:
  VINP_BrkSwSta_flg/1 -> [VINP_BrkSwSta_flg]
  VTQD_AfterAvailableTqDemFr_Nm/1 -> [VTQD_AfterAvailableTqDemFr_Nm]
  [VVMC_RF4WhlSpdSlideRate_pct] -> VVMC_RF4WhlSpdSlideRate_pct/1
  [VVMC_ActRRSlideRate_pct] -> VVMC_ActRRSlideRate_pct/1
  VTQD_EquivAccPedalSWSta_flg/1 -> [VTQD_EquivAccPedalSWSta_flg]
  [VVMC_LFWhlSpdSlideRate_pct] -> VVMC_LFWhlSpdSlideRate_pct/1
  VINP_BrkPedalPos_pct/1 -> [VINP_BrkPedalPos_pct]
  [VVMC_RRWhlSpdSlideRate_pct] -> VVMC_RRWhlSpdSlideRate_pct/1
  task_time_s/1 -> [task_time_s]
  VINP_RRRawWhlSpeed_kph/1 -> [VINP_RRRawWhlSpeed_kph]
  [VVMC_ActMaxSlideRate_pct] -> VVMC_ActMaxSlideRate_pct/1
  [VVMC_RFWhlSpdSlideRate_pct] -> VVMC_RFWhlSpdSlideRate_pct/1
  [VVMC_LR4WhlSpdSlideRate_pct] -> VVMC_LR4WhlSpdSlideRate_pct/1
  [VVMC_ActRFSlideRate_pct] -> VVMC_ActRFSlideRate_pct/1
  [VVMC_RR4WhlSpdSlideRate_pct] -> VVMC_RR4WhlSpdSlideRate_pct/1
  VINP_RFRawWhlSpeed_kph/1 -> [VINP_RFRawWhlSpeed_kph]
  VINP_VehSpeed_kph/1 -> [VINP_VehSpeed_kph]
  [VVMC_ActLRSlideRate_pct] -> VVMC_ActLRSlideRate_pct/1
  [VVMC_PredictVehSpd_kph] -> VVMC_PredictVehSpd_kph/1
  VINP_LRRawWhlSpeed_kph/1 -> [VINP_LRRawWhlSpeed_kph]
  [VVMC_LF4WhlSpdSlideRate_pct] -> VVMC_LF4WhlSpdSlideRate_pct/1
  [VVMC_RawWhlSpdSlideRate_pct] -> VVMC_RawWhlSpdSlideRate_pct/1
  VINP_LFRawWhlSpeed_kph/1 -> [VINP_LFRawWhlSpeed_kph]
  [VVMC_LRWhlSpdSlideRate_pct] -> VVMC_LRWhlSpdSlideRate_pct/1
  [VVMC_ActLFSlideRate_pct] -> VVMC_ActLFSlideRate_pct/1
  [VVMC_4WhlSpdSlideRate_pct] -> VVMC_4WhlSpdSlideRate_pct/1
  VVMC_LongAcc_Gps/1 -> [VVMC_LongAcc_Gps]
  VTQD_AfterAvailableTqDemRr_Nm/1 -> [VTQD_AfterAvailableTqDemRr_Nm]
  [VINP_LFRawWhlSpeed_kph] -> Alternative Wheel Slide Calculation/1(VINP_LFRawWhlSpeed_kph)
  [VINP_RFRawWhlSpeed_kph] -> Alternative Wheel Slide Calculation/2(VINP_RFRawWhlSpeed_kph)
  [VINP_LRRawWhlSpeed_kph] -> Alternative Wheel Slide Calculation/3(VINP_LRRawWhlSpeed_kph)
  [VINP_RRRawWhlSpeed_kph] -> Alternative Wheel Slide Calculation/4(VINP_RRRawWhlSpeed_kph)
  Alternative Wheel Slide Calculation/1(VVMC_AltLWhlSlideRate_pct) -> [VVMC_AltLWhlSlideRate_pct]
  Alternative Wheel Slide Calculation/2(VVMC_AltRWhlSlideRate_pct) -> [VVMC_AltRWhlSlideRate_pct]
  Alternative Wheel Slide Calculation/3(VVMC_AltWhlSlideRate_pct) -> [VVMC_AltWhlSlideRate_pct]
  [VVMC_AltLWhlSlideRate_pct] -> VVMC_AltLWhlSlideRate_pct/1
  [VVMC_AltRWhlSlideRate_pct] -> VVMC_AltRWhlSlideRate_pct/1
  [VVMC_AltWhlSlideRate_pct] -> VVMC_AltWhlSlideRate_pct/1
  Partial Wheel Calculation/2(VVMC_LFWhlSpdSlideRate_pct) -> [VVMC_LFWhlSpdSlideRate_pct]
  Partial Wheel Calculation/5(VVMC_RRWhlSpdSlideRate_pct) -> [VVMC_RRWhlSpdSlideRate_pct]
  Partial Wheel Calculation/3(VVMC_RFWhlSpdSlideRate_pct) -> [VVMC_RFWhlSpdSlideRate_pct]
  Partial Wheel Calculation/1(VVMC_RawWhlSpdSlideRate_pct) -> [VVMC_RawWhlSpdSlideRate_pct]
  [VINP_RFRawWhlSpeed_kph] -> Partial Wheel Calculation/2(VINP_RFRawWhlSpeed_kph)
  [VINP_LRRawWhlSpeed_kph] -> Partial Wheel Calculation/3(VINP_LRRawWhlSpeed_kph)
  [VTQD_AfterAvailableTqDemFr_Nm] -> Partial Wheel Calculation/5(VTQD_AfterAvailableTqDemFr_Nm)
  [VINP_LFRawWhlSpeed_kph] -> Partial Wheel Calculation/1(VINP_LFRawWhlSpeed_kph)
  [VINP_RRRawWhlSpeed_kph] -> Partial Wheel Calculation/4(VINP_RRRawWhlSpeed_kph)
  [VTQD_AfterAvailableTqDemRr_Nm] -> Partial Wheel Calculation/6(VTQD_AfterAvailableTqDemRr_Nm)
  Partial Wheel Calculation/4(VVMC_LRWhlSpdSlideRate_pct) -> [VVMC_LRWhlSpdSlideRate_pct]
  4Wheel Calculation/3(VVMC_LR4WhlSpdSlideRate_pct) -> [VVMC_LR4WhlSpdSlideRate_pct]
  [task_time_s] -> 4Wheel Calculation/6(task_time_s)
  4Wheel Calculation/1(VVMC_LF4WhlSpdSlideRate_pct) -> [VVMC_LF4WhlSpdSlideRate_pct]
  4Wheel Calculation/7(VVMC_AllWhlSkid_flg) -> [VVMC_AllWhlSkid_flg]
  [VVMC_LongAcc_Gps] -> 4Wheel Calculation/5(VVMC_LongAcc_Gps)
  4Wheel Calculation/4(VVMC_RR4WhlSpdSlideRate_pct) -> [VVMC_RR4WhlSpdSlideRate_pct]
  [VTQD_AfterAvailableTqDemRr_Nm] -> 4Wheel Calculation/9(VTQD_AfterAvailableTqDemRr_Nm)
  [VTQD_AfterAvailableTqDemFr_Nm] -> 4Wheel Calculation/8(VTQD_AfterAvailableTqDemFr_Nm)
  [VINP_VehSpeed_kph] -> 4Wheel Calculation/7(VINP_VehSpeed_kph)
  4Wheel Calculation/5(VVMC_PredictVehSpd_kph) -> [VVMC_PredictVehSpd_kph]
  [VINP_LRRawWhlSpeed_kph] -> 4Wheel Calculation/3(VINP_LRRawWhlSpeed_kph)
  [VINP_RRRawWhlSpeed_kph] -> 4Wheel Calculation/4(VINP_RRRawWhlSpeed_kph)
  [VINP_LFRawWhlSpeed_kph] -> 4Wheel Calculation/1(VINP_LFRawWhlSpeed_kph)
  [VINP_RFRawWhlSpeed_kph] -> 4Wheel Calculation/2(VINP_RFRawWhlSpeed_kph)
  4Wheel Calculation/2(VVMC_RF4WhlSpdSlideRate_pct) -> [VVMC_RF4WhlSpdSlideRate_pct]
  4Wheel Calculation/6(VVMC_4WhlSpdSlideRate_pct) -> [VVMC_4WhlSpdSlideRate_pct]
  [VVMC_LF4WhlSpdSlideRate_pct] -> Coordination/14(VVMC_LF4WhlSpdSlideRate_pct)
  [VVMC_RR4WhlSpdSlideRate_pct] -> Coordination/17(VVMC_RR4WhlSpdSlideRate_pct)
  [VVMC_LR4WhlSpdSlideRate_pct] -> Coordination/16(VVMC_LR4WhlSpdSlideRate_pct)
  [task_time_s] -> Coordination/6(task_time_s)
  [VVMC_LFWhlSpdSlideRate_pct] -> Coordination/9(VVMC_LFWhlSpdSlideRate_pct)
  [VTQD_AfterAvailableTqDemFr_Nm] -> Coordination/1(VTQD_AfterAvailableTqDemFr_Nm)
  [VVMC_AltWhlSlideRate_pct] -> Coordination/20(VVMC_AltWhlSlideRate_pct)
  [VVMC_RFWhlSpdSlideRate_pct] -> Coordination/10(VVMC_RFWhlSpdSlideRate_pct)
  [VTQD_EquivAccPedalSWSta_flg] -> Coordination/2(VTQD_EquivAccPedalSWSta_flg)
  [VVMC_AllWhlSkid_flg] -> Coordination/18(VVMC_AllWhlSkid_flg)
  [VVMC_4WhlSpdSlideRate_pct] -> Coordination/13(VVMC_4WhlSpdSlideRate_pct)
  [VINP_VehSpeed_kph] -> Coordination/5(VINP_VehSpeed_kph)
  Coordination/3(VVMC_ActRFSlideRate_pct) -> [VVMC_ActRFSlideRate_pct]
  [VVMC_RawWhlSpdSlideRate_pct] -> Coordination/8(VVMC_RawWhlSpdSlideRate_pct)
  [VTQD_AfterAvailableTqDemRr_Nm] -> Coordination/19(VTQD_AfterAvailableTqDemRr_Nm)
  Coordination/4(VVMC_ActLRSlideRate_pct) -> [VVMC_ActLRSlideRate_pct]
  [VVMC_PredictVehSpd_kph] -> Coordination/4(VVMC_PredictVehSpd_kph)
  [VINP_BrkSwSta_flg] -> Coordination/7(VINP_BrkSwSta_flg)
  [VVMC_LRWhlSpdSlideRate_pct] -> Coordination/11(VVMC_LRWhlSpdSlideRate_pct)
  [VVMC_RRWhlSpdSlideRate_pct] -> Coordination/12(VVMC_RRWhlSpdSlideRate_pct)
  [VINP_BrkPedalPos_pct] -> Coordination/3(VINP_BrkPedalPos_pct)
  Coordination/1(VVMC_ActMaxSlideRate_pct) -> [VVMC_ActMaxSlideRate_pct]
  Coordination/5(VVMC_ActRRSlideRate_pct) -> [VVMC_ActRRSlideRate_pct]
  Coordination/2(VVMC_ActLFSlideRate_pct) -> [VVMC_ActLFSlideRate_pct]
  [VVMC_RF4WhlSpdSlideRate_pct] -> Coordination/15(VVMC_RF4WhlSpdSlideRate_pct)
  [VTQD_GearActualPosn_enum] -> 4Wheel Calculation/10(VTQD_GearActualPosn_enum)
  VTQD_GearActualPosn_enum/1 -> [VTQD_GearActualPosn_enum]
  VINP_LongAccel_Gps/1 -> [VINP_LongAccel_Gps]
  [VINP_LongAccel_Gps] -> 4Wheel Calculation/11(VINP_LongAccel_Gps)

== system vmc/VMC/VMC/SpeedArbitration ==
  VVMC_VMCCCCtrlAvail_flg : Inport
  VVMC_VMCMSACtrlAvail_flg : Inport  Port=2
  VVMC_VMCACCCtrlAvail_flg : Inport  Port=3
  VVMC_VMCAEBCtrlAvail_flg : Inport  Port=4
  VINP_ADASAEBReq_enum : Inport  Port=5
  VINP_ADASAEBSta_enum : Inport  Port=6
  VDSC_DISCSta_enum : Inport  Port=7
  VINP_ADASACCSta_enum : Inport  Port=8
  VVMC_CCCtrlSta_enum : Inport  Port=9
  VVMC_MSACtrlSta_enum : Inport  Port=10
  VDSC_DISCTargetSpd_kph : Inport  Port=11
  VVMC_FeatSetSpdForCalcu_kph : Inport  Port=12
  VDSC_DISCTurn_flg : Inport  Port=13
  VVMC_MeterIndSpeedForCalcu_kph : Inport  Port=14
  VINP_VehSpeed_kph : Inport  Port=15
  VVMC_LastFeatArbitrFinal_enum : Inport  Port=16
  VVMC_LastActACCRequiredAccel_mps2 : Inport  Port=17
  VDSC_AccDecResp_flg : Inport  Port=18
  VDSC_AutoTurnMode_flg : Inport  Port=19
  VVMC_AntiSpdLimEn_flg : Inport  Port=20
  Cast To Single : DataTypeConversion  OutDataTypeStr=uint8
  Cast To Single1 : DataTypeConversion  OutDataTypeStr=uint8
  Cast To Single2 : DataTypeConversion  OutDataTypeStr=single
  Cast To Single3 : DataTypeConversion  OutDataTypeStr=single
  Cast To Single4 : DataTypeConversion  OutDataTypeStr=single
  Constant : Constant  Value=KVMC_ExternalCtrlSW_flg
  Constant1 : Constant  Value=KVMC_ExternalCtrlSW_flg
  Constant10 : Constant  Value=KVMC_AntiSpdLim_kph
  Constant2 : Constant  Value=KVMC_ExternalCtrlSW_flg
  Constant3 : Constant  Value=KVMC_ExternalCtrlSta_enum
  Constant4 : Constant  Value=KVMC_ExternalSpeedTarget_kph
  Constant5 : Constant  Value=KVMC_ExternalCtrlAGSV_flg
  Constant6 : Constant  Value=KVMC_AutoTurnJerkHiGain_pct
  Constant7 : Constant  Value=KVMC_AutoTurnLimitHiGain_pct
  Constant8 : Constant  Value=ENUM_FEATSTACFM_MSA
  Constant9 : Constant  Value=ENUM_FEATSTACFM_MSA
  Divide : Product  Inputs=**
  Divide1 : Product  Inputs=**
  Feature Arbitration : Subsystem
  Feature Status Confirm : Subsystem
  Response Gain : Subsystem
  Round : Rounding  Operator=round
  Switch{,1..7} (8 alike) : Switch  Criteria=u2 > Threshold
  VVMC_FeatArbitrSta_enum : Outport
  VVMC_FeatReqSpd_kph : Outport  Port=2
  VVMC_JerkPCT_pct : Outport  Port=3
  VVMC_LimitPCT_pct : Outport  Port=4
  wires:
  [VINP_VehSpeed_kph] -> Response Gain/5(VINP_VehSpeed_kph)
  VINP_VehSpeed_kph/1 -> [VINP_VehSpeed_kph]
  [VVMC_FeatReqSpd_kph] -> Response Gain/3(VVMC_FeatReqSpd_kph)
  [VVMC_MeterIndSpeedForCalcu_kph] -> Response Gain/4(VVMC_MeterIndSpeedForCalcu_kph)
  VVMC_MeterIndSpeedForCalcu_kph/1 -> [VVMC_MeterIndSpeedForCalcu_kph]
  Round/1 -> Cast To Single2/1
  [VINP_ADASAEBReq_enum] -> Feature Status Confirm/10(VINP_ADASAEBReq_enum)
  VINP_ADASAEBReq_enum/1 -> [VINP_ADASAEBReq_enum]
  [VVMC_VMCCCCtrlAvail_flg] -> Feature Status Confirm/1(VVMC_VMCCCCtrlAvail_flg)
  [VVMC_VMCMSACtrlAvail_flg] -> Feature Status Confirm/2(VVMC_VMCMSACtrlAvail_flg)
  VVMC_VMCCCCtrlAvail_flg/1 -> [VVMC_VMCCCCtrlAvail_flg]
  VVMC_VMCMSACtrlAvail_flg/1 -> [VVMC_VMCMSACtrlAvail_flg]
  [VVMC_VMCAEBCtrlAvail_flg] -> Feature Status Confirm/3(VVMC_VMCAEBCtrlAvail_flg)
  [VVMC_VMCACCCtrlAvail_flg] -> Feature Status Confirm/4(VVMC_VMCACCCtrlAvail_flg)
  VVMC_VMCAEBCtrlAvail_flg/1 -> [VVMC_VMCAEBCtrlAvail_flg]
  VVMC_VMCACCCtrlAvail_flg/1 -> [VVMC_VMCACCCtrlAvail_flg]
  Switch4/1 -> [VVMC_LimitPCT_pct]  "VVMC_LimitPCT_pct"
  Switch3/1 -> [VVMC_JerkPCT_pct]  "VVMC_JerkPCT_pct"
  Switch7/1 -> [VVMC_FeatReqSpd_kph]  "VVMC_FeatReqSpd_kph"
  Switch6/1 -> [VVMC_FeatArbitrSta_enum]  "VVMC_FeatArbitrSta_enum"
  Switch5/1 -> [VVMC_FeatStaConfirm_enum]  "VVMC_FeatStaConfirm_enum"
  [VVMC_JerkPCT_pct] -> VVMC_JerkPCT_pct/1
  [VVMC_LimitPCT_pct] -> VVMC_LimitPCT_pct/1
  Response Gain/1(VVMC_JerkPCT_pct) -> Cast To Single3/1
  Response Gain/2(VVMC_LimitPCT_pct) -> Cast To Single4/1
  [VVMC_FeatArbitrSta_enum] -> Response Gain/2(VVMC_FeatArbitrSta_enum)
  Switch2/1 -> Response Gain/1(VDSC_DISCTurn_flg)
  [VVMC_FeatReqSpd_kph] -> VVMC_FeatReqSpd_kph/1
  [VVMC_FeatArbitrSta_enum] -> VVMC_FeatArbitrSta_enum/1
  Feature Arbitration/2(VVMC_FeatReqSpd_kph) -> Round/1
  Feature Arbitration/1(VVMC_FeatArbitrSta_enum) -> Cast To Single1/1
  [VVMC_FeatSetSpdForCalcu_kph] -> Feature Arbitration/3(VVMC_FeatSetSpdForCalcu_kph)
  [VVMC_FeatStaConfirm_enum] -> Feature Arbitration/1(VVMC_FeatStaConfirm_enum)
  Feature Status Confirm/1(VVMC_FeatStaConfirm_enum) -> Cast To Single/1
  [VVMC_MSACtrlSta_enum] -> Feature Status Confirm/9(VVMC_MSACtrlSta_enum)
  [VVMC_CCCtrlSta_enum] -> Feature Status Confirm/8(VVMC_CCCtrlSta_enum)
  [VINP_ADASACCSta_enum] -> Feature Status Confirm/7(VINP_ADASACCSta_enum)
  Switch/1 -> Feature Status Confirm/6(VDSC_DISCSta_enum)
  [VINP_ADASAEBSta_enum] -> Feature Status Confirm/5(VINP_ADASAEBSta_enum)
  VDSC_DISCTurn_flg/1 -> [VDSC_DISCTurn_flg]
  VVMC_FeatSetSpdForCalcu_kph/1 -> [VVMC_FeatSetSpdForCalcu_kph]
  VDSC_DISCTargetSpd_kph/1 -> [VDSC_DISCTargetSpd_kph]
  VVMC_MSACtrlSta_enum/1 -> [VVMC_MSACtrlSta_enum]
  VVMC_CCCtrlSta_enum/1 -> [VVMC_CCCtrlSta_enum]
  VINP_ADASACCSta_enum/1 -> [VINP_ADASACCSta_enum]
  VDSC_DISCSta_enum/1 -> [VDSC_DISCSta_enum]
  VINP_ADASAEBSta_enum/1 -> [VINP_ADASAEBSta_enum]
  Switch1/1 -> Feature Arbitration/2(VDSC_DISCTargetSpd_kph)
  [VDSC_DISCSta_enum] -> Switch/3
  Constant1/1 -> Switch1/2
  Constant5/1 -> Switch2/1
  [VDSC_DISCTargetSpd_kph] -> Switch1/3
  Constant3/1 -> Switch/1
  Constant2/1 -> Switch2/2
  Constant4/1 -> Switch1/1
  Constant/1 -> Switch/2
  [VDSC_DISCTurn_flg] -> Switch2/3
  VVMC_LastFeatArbitrFinal_enum/1 -> [VVMC_LastFeatArbitrFinal_enum]
  VVMC_LastActACCRequiredAccel_mps2/1 -> [VVMC_LastActACCRequiredAccel_mps2]
  [VVMC_LastFeatArbitrFinal_enum] -> Feature Arbitration/4(VVMC_LastFeatArbitrFinal_enum)
  [VVMC_LastActACCRequiredAccel_mps2] -> Feature Arbitration/5(VVMC_LastActACCRequiredAccel_mps2)
  VDSC_AccDecResp_flg/1 -> [VDSC_AccDecResp_flg]
  [VDSC_AccDecResp_flg] -> Switch3/2
  Cast To Single3/1 -> Switch3/3, Divide/2
  Constant6/1 -> Divide/1
  Divide/1 -> Switch3/1
  Divide1/1 -> Switch4/1
  Constant7/1 -> Divide1/1
  Cast To Single4/1 -> Divide1/2, Switch4/3
  [VDSC_AccDecResp_flg] -> Switch4/2
  VDSC_AutoTurnMode_flg/1 -> [VDSC_AutoTurnMode_flg]
  [VDSC_AutoTurnMode_flg] -> Response Gain/6(VDSC_AutoTurnMode_flg)
  VVMC_AntiSpdLimEn_flg/1 -> [VVMC_AntiSpdLimEn_flg]
  [VVMC_AntiSpdLimEn_flg] -> Switch5/2
  Cast To Single/1 -> Switch5/3
  Constant8/1 -> Switch5/1
  Constant9/1 -> Switch6/1
  [VVMC_AntiSpdLimEn_flg] -> Switch6/2
  Cast To Single1/1 -> Switch6/3
  [VVMC_AntiSpdLimEn_flg] -> Switch7/2
  Cast To Single2/1 -> Switch7/3
  Constant10/1 -> Switch7/1
